simulink model "motor_cooling"  (R2021a)
settings: Solver=FixedStepAuto  StartTime=0.0  StopTime=Tsim  FixedStep=1  RelTol=1e-3
values from neighbouring files (symbols this model uses):
  Cm = Motor_cooling_max_power/(Cp*(Tm_at_max_HP-Tamb))    [imports_motor_cooling.m]
  Cp = 1350    [imports_motor_cooling.m]
  mCp = 1350    [imports_motor_cooling.m]
  Mm = 23.69    [imports_motor_cooling.m]
  Tamb = 293.15    [imports_battery_cooling.m]    (also in imports_motor_cooling.m = 18)
  Tmotor_i = 20    [imports_motor_cooling.m]
settings Model: Creator=shubh  LastModifiedBy=shubh

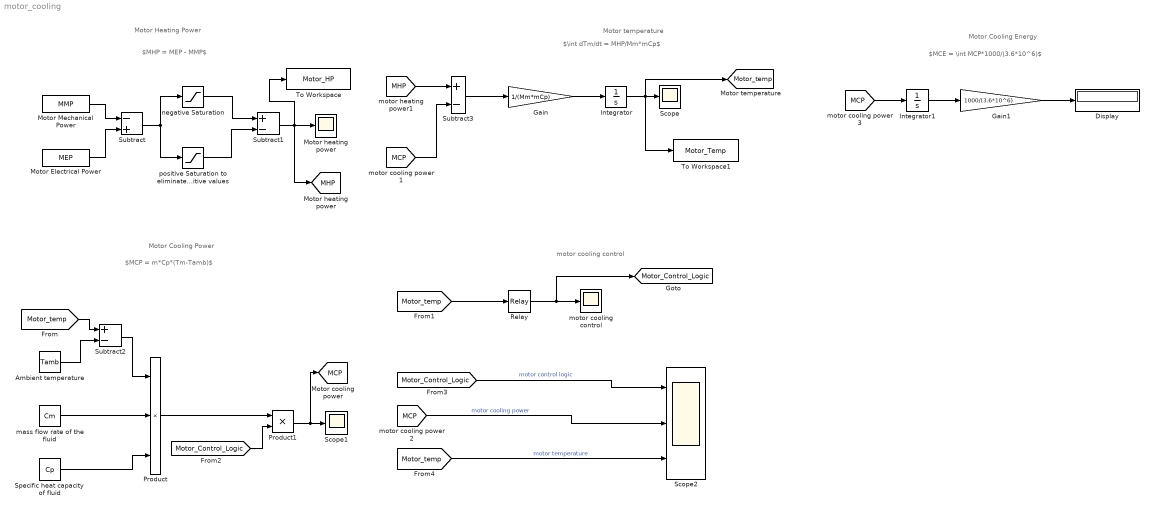
== system motor_cooling ==
  note: Motor Cooling Energy
  note: $MCE = \int MCP*1000/(3.6*10^6)$
  note: motor cooling control
  note: Motor Cooling Power
  note: $MCP = m*Cp*(Tm-Tamb)$
  note: $\int dTm/dt = MHP/Mm*mCp$
  note: Motor temperature
  note: $MHP = MEP - MMP$
  note: Motor Heating Power
  Ambient temperature : Constant  Value=Tamb
  Display : Display
  Gain : Gain  Gain=1/(Mm*mCp)
  Gain1 : Gain  Gain=1000/(3.6*10^6)
  Integrator : Integrator  InitialCondition=Tmotor_i
  Integrator1 : Integrator
  Motor Electrical Power : FromWorkspace  VariableName=MEP
  Motor Mechanical Power : FromWorkspace  VariableName=MMP
  Motor heating power : Scope
  Product : Product  Inputs=3
  Product1 : Product
  Relay : Relay  OnSwitchValue=30  OffSwitchValue=20
  Scope : Scope
  Scope1 : Scope
  Scope2 : Scope  NumInputPorts=3
  Specific heat capacity of fluid : Constant  Value=Cp
  Subtract : Sum  Inputs=-+
  Subtract1 : Sum  Inputs=+-
  Subtract2 : Sum  Inputs=+-
  Subtract3 : Sum  Inputs=+-
  To Workspace : ToWorkspace  VariableName=Motor_HP  SaveFormat=Timeseries  SampleTime=-1
  To Workspace1 : ToWorkspace  VariableName=Motor_Temp  SaveFormat=Timeseries  SampleTime=-1
  mass flow rate of the fluid : Constant  Value=Cm
  motor cooling control : Scope
  negative Saturation : Saturate  UpperLimit=inf  LowerLimit=0
  positive Saturation to eliminate positive values : Saturate  UpperLimit=0  LowerLimit=-inf
  tag scope: MCP=global, MHP=global, Motor_Control_Logic=global, Motor_temp=global
  wires:
  Motor Mechanical Power/1 -> Subtract/1
  Motor Electrical Power/1 -> Subtract/2
  Subtract/1 -> positive Saturation to eliminate positive values/1, negative Saturation/1
  positive Saturation to eliminate positive values/1 -> Subtract1/2
  negative Saturation/1 -> Subtract1/1
  Subtract1/1 -> To Workspace/1, [MHP], Motor heating power/1
  Integrator/1 -> [Motor_temp], To Workspace1/1, Scope/1
  Gain/1 -> Integrator/1
  [Motor_temp] -> Subtract2/1
  Ambient temperature/1 -> Subtract2/2
  Subtract2/1 -> Product/1
  mass flow rate of the fluid/1 -> Product/2
  Specific heat capacity of fluid/1 -> Product/3
  [MHP] -> Subtract3/1
  Subtract3/1 -> Gain/1
  [MCP] -> Subtract3/2
  [Motor_temp] -> Relay/1
  Relay/1 -> [Motor_Control_Logic], motor cooling control/1
  Product1/1 -> [MCP], Scope1/1
  [Motor_Control_Logic] -> Product1/2
  Product/1 -> Product1/1
  [Motor_Control_Logic] -> Scope2/1  "motor control logic"
  [MCP] -> Scope2/2  "motor cooling power"
  [Motor_temp] -> Scope2/3  "motor temperature"
  [MCP] -> Integrator1/1
  Integrator1/1 -> Gain1/1
  Gain1/1 -> Display/1
